simulink model "pfc_desktop_hdl"  (R2024b)
settings: Solver=FixedStepDiscrete  StartTime=0.0  StopTime=.4  RelTol=1e-3
InitFcn:
  | fidelity_pfc_vals;
values from neighbouring files (symbols this model uses):
  fsw = 65    [fidelity_pfc_vals.m]
  Gs = 2e-2    (= 0.02)    [fidelity_pfc_vals.m]
  s = 1    [fidelity_pfc_vals.m]
  t_ss = tsw/30    (= 5.12820512821e-07)    [fidelity_pfc_vals.m]
  tsw = 1/(fsw*1e3)    (= 1.53846153846e-05)    [fidelity_pfc_vals.m]
undefined symbols (not defined in the file or in its folder): a, b, c, DiscIntNeverNeededParam
libraries: fl_lib x37, nesl_utility x31, hdlsllib x6, mcbcontrolslib x5, ee_lib x5, dspsrcs4 x3, slpidlib x2, simulink x1, spsSVPWMGenerator2LevelLib x1, spsPLL3phLib x1
(part 2 of 2)

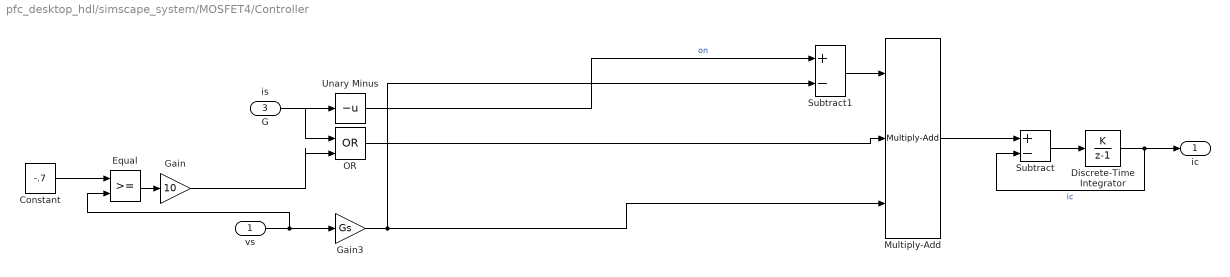
== system pfc_desktop_hdl/simscape_system/MOSFET4/Controller ==
  vs : Inport
  is : Inport  Port=2
  G : Inport  Port=3
  Constant : Constant  Value=-.7  SampleTime=-1
  Discrete-Time Integrator : DiscreteIntegrator  IntegratorMethod=Accumulation: Forward Euler  gainval=1/s  SampleTime=-1  OutDataTypeStr=Inherit: Inherit via back propagation  ICPrevOutput=DiscIntNeverNeededParam  ICPrevScaledInput=DiscIntNeverNeededParam
  Equal : RelationalOperator  OutDataTypeStr=boolean  RndMeth=Simplest  InputSameDT=off
  Gain : Gain  Gain=10
  Gain3 : Gain  Gain=Gs  OutDataTypeStr=Inherit: Inherit via back propagation
  Multiply-Add : hdlsllib/HDL Operations/Multiply-Add  Function=c+(a.*b)  datatype=Inherit: Inherit via internal rule  DoSatur=off  FMA=off
  OR : Logic  Operator=OR  IconShape=distinctive  AllPortsSameDT=off  OutDataTypeStr=boolean
  Subtract : Sum  Inputs=+-
  Subtract1 : Sum  Inputs=+-
  Unary Minus : UnaryMinus
  ic : Outport
  wires:
  OR/1 -> Multiply-Add/2
  Subtract1/1 -> Multiply-Add/1
  Gain3/1 -> Multiply-Add/3, Subtract1/2
  Constant/1 -> Equal/1
  Gain/1 -> OR/2
  Equal/1 -> Gain/1
  vs/1 -> Gain3/1, Equal/2
  Subtract/1 -> Discrete-Time Integrator/1
  Discrete-Time Integrator/1 -> Subtract/2, ic/1  "ic"
  is/1 -> Unary Minus/1
  Unary Minus/1 -> Subtract1/1  "on"
  G/1 -> OR/1
  Multiply-Add/1 -> Subtract/1

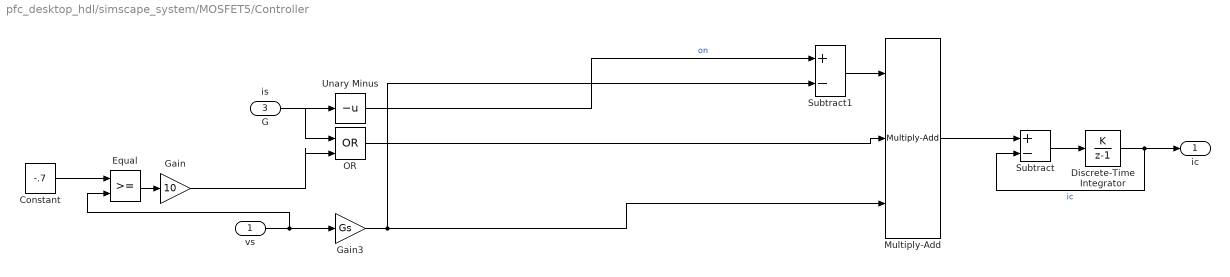
== system pfc_desktop_hdl/simscape_system/MOSFET5/Controller ==
  vs : Inport
  is : Inport  Port=2
  G : Inport  Port=3
  Constant : Constant  Value=-.7  SampleTime=-1
  Discrete-Time Integrator : DiscreteIntegrator  IntegratorMethod=Accumulation: Forward Euler  gainval=1/s  SampleTime=-1  OutDataTypeStr=Inherit: Inherit via back propagation  ICPrevOutput=DiscIntNeverNeededParam  ICPrevScaledInput=DiscIntNeverNeededParam
  Equal : RelationalOperator  OutDataTypeStr=boolean  RndMeth=Simplest  InputSameDT=off
  Gain : Gain  Gain=10
  Gain3 : Gain  Gain=Gs  OutDataTypeStr=Inherit: Inherit via back propagation
  Multiply-Add : hdlsllib/HDL Operations/Multiply-Add  Function=c+(a.*b)  datatype=Inherit: Inherit via internal rule  DoSatur=off  FMA=off
  OR : Logic  Operator=OR  IconShape=distinctive  AllPortsSameDT=off  OutDataTypeStr=boolean
  Subtract : Sum  Inputs=+-
  Subtract1 : Sum  Inputs=+-
  Unary Minus : UnaryMinus
  ic : Outport
  wires:
  Multiply-Add/1 -> Subtract/1
  G/1 -> OR/1
  Unary Minus/1 -> Subtract1/1  "on"
  is/1 -> Unary Minus/1
  Discrete-Time Integrator/1 -> ic/1, Subtract/2  "ic"
  Subtract/1 -> Discrete-Time Integrator/1
  vs/1 -> Equal/2, Gain3/1
  Equal/1 -> Gain/1
  Gain/1 -> OR/2
  Constant/1 -> Equal/1
  Gain3/1 -> Subtract1/2, Multiply-Add/3
  Subtract1/1 -> Multiply-Add/1
  OR/1 -> Multiply-Add/2

== system pfc_desktop_hdl/Subsystem1/ctrl_pwm/transforms/Claro-Parl Transform ==
  a : Inport
  b : Inport  Port=2
  wt : Inport  Port=3
  Clarke Transform : mcbcontrolslib/Clarke Transform  VariantControl=Variant2  PhaseInput=Two inputs  EnPowerInv=off
  Cos : Trigonometry  Operator=cos
  Park Transform : mcbcontrolslib/Park Transform  PhaseInput=Two inputs  AxisAlignment=D-axis  ThetaInput=Sine and Cosine electrical position  AngleInput=Per-unit  N_points=1024
  Sin : Trigonometry
  d : Outport
  q : Outport  Port=2
  wires:
  Clarke Transform/2 -> Park Transform/2  "Vbet_sourc"
  b/1 -> Clarke Transform/2
  Park Transform/2 -> q/1
  Park Transform/1 -> d/1
  Clarke Transform/1 -> Park Transform/1  "Valp_sourc"
  wt/1 -> Cos/1, Sin/1
  a/1 -> Clarke Transform/1
  Sin/1 -> Park Transform/3
  Cos/1 -> Park Transform/4

== system pfc_desktop_hdl/Subsystem1/ctrl_pwm/transforms/Claro-Parl Transform1 ==
  a : Inport
  b : Inport  Port=2
  wt : Inport  Port=3
  Clarke Transform : mcbcontrolslib/Clarke Transform  VariantControl=Variant2  PhaseInput=Two inputs  EnPowerInv=off
  Cos : Trigonometry  Operator=cos
  Park Transform : mcbcontrolslib/Park Transform  PhaseInput=Two inputs  AxisAlignment=D-axis  ThetaInput=Sine and Cosine electrical position  AngleInput=Per-unit  N_points=1024
  Sin : Trigonometry
  d : Outport
  q : Outport  Port=2
  wires:
  Clarke Transform/2 -> Park Transform/2  "Ibet_sourc"
  b/1 -> Clarke Transform/2
  Park Transform/2 -> q/1
  Park Transform/1 -> d/1
  Clarke Transform/1 -> Park Transform/1  "Ialp_sourc"
  wt/1 -> Cos/1, Sin/1
  a/1 -> Clarke Transform/1
  Sin/1 -> Park Transform/3
  Cos/1 -> Park Transform/4
